simulink model "svm_test"  (Simulink 8.6)
settings: Solver=ode1  StartTime=0.0  StopTime=svm.tsim  FixedStep=uavsim.svm.tsample_model  RelTol=1e-3
values from neighbouring files (symbols this model uses):
  uavsim = loaded.uavsim    [svm_sandbox.m]
undefined symbols (not defined in the file or in its folder): svm
libraries: dspsrcs4 x2, aerolibtransform2 x2, aerolibanimutils x1, svm_lib x1, uavsimBlockset_UAV3DInterface x1
settings Model: Creator=j.bolting  LastModifiedBy=j.bolting
settings SolverCC: AutoInsertRateTranBlk=on
settings DataIOCC: SaveFormat=Dataset  SignalLoggingSaveFormat=Dataset
settings OptimizationCC: ExpressionDepthLimit=128
settings DebuggingCC: UnderspecifiedInitializationDetection=Simplified  MergeDetectMultiDrivingBlocksExec=error  SolverPrmCheckMsg=none  FcnCallInpInsideContextMsg=EnableAllAsError  StateNameClashWarn=none
settings HardwareCC: ProdBitPerPointer=64  ProdLargestAtomicFloat=Float  ProdIntDivRoundTo=Zero  ProdEndianess=LittleEndian  ProdWordSize=64  ProdHWDeviceType=Intel->x86-64 (Windows64)
settings GRTTargetCC: GeneratePreprocessorConditionals=Use local settings  CombineOutputUpdateFcns=on  GRTInterface=off
settings ConfigComp: CovModelRefEnable=off

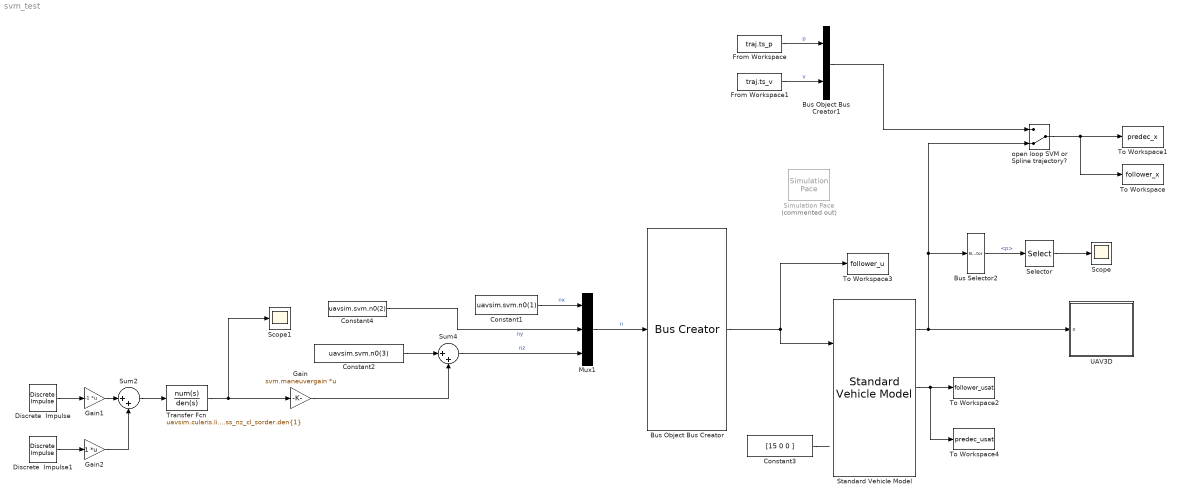
== system svm_test ==
  Bus Selector2 : BusSelector  OutputSignals=p
  Bus Object Bus Creator : BusCreator  Inputs=1  OutDataTypeStr=Bus: svm_bus_u  mask(BUS OBJECT Bus Creator){busType=Bus: svm_bus_u}
      mask prompts: busType "Bus Type"
      mask help:
      | Provides users the cabability to painlessly, instantly customize bus creators of output data type 'Bus:' by selecting the bus object type from a drop down menu dynamically populated by bus objects in the workspace.
      |
      | After pressing the "Apply Selection" button signal lines into the creator are populated and named with the elements in the chosen bus saving the user from having to recall and fill out signal line names.
      |
      | NOTE that when copying a Bus Object Bus Creator from your locked Library the link to the Library is automatically broken. This saves the user from having to Unlock Links To Library (From the Library menu.), Disable Link and finally Break Link (Both from the Model menu.) for every placed instance of the block.
      settings: AttributesFormatString=%<OutDataTypeStr>  CopyFcn=set_param(gcb, 'LinkStatus', 'none')
      mask TypeOptions busType: Bus: Acceleration | Bus: Aero | Bus: Airframe | Bus: Attitude | Bus: CMD | Bus: Environment | Bus: FlightGearData | Bus: Kinematics | Bus: Position | Bus: RotationalAcceleration | Bus: RotationalVelocity | Bus: Velocity | Bus: svm_bus_d_exo | Bus: svm_bus_u | Bus: svm_bus_x | Bus: svm_bus_xi
      mask Callback busType:
      | % Using variable names terminated with "_BOBC" to lessen the chances of
      | % collisions with existing workspace variables.
      | 
      | % Get the current block handle and mask handle.
      | handleCreator_BOBC = gcbh;
      | maskObj_BOBC       = Simulink.Mask.get(gcb);
      | 
      | % Get a list of variables in the workspace in order to search for the '1x1
      | % Bus' types.
      | wsVars_BOBC = whos;
      | 
      | % Reset the 'TypeOptions' bus list in case some '1x1 Bus' types have been
      | % deleted from or added to the workspace.
      | maskObj_BOBC.Parameters.TypeOptions = {'<empty>'};
      | 
      | % Reset the bus count.
      | busCount_BOBC = 0;
      | 
      | for index_BOBC = 1:length(wsVars_BOBC)
      | 
      |    % If the variable is a bus object...
      |    if strcmp(wsVars_BOBC(index_BOBC).class, 'Simulink.Bus')
      | 
      |       busCount_BOBC = busCount_BOBC + 1;
      | 
      |       % ... add it to the TypeOptions of the mask.
      |       maskObj_BOBC.Parameters.TypeOptions(busCount_BOBC) = ...
      |                                                            ...
      |                                  {['Bus: ', wsVars_BOBC(index_BOBC).name]};
      |    end
      | end
      | 
      | if busCount_BOBC == 0
      | 
      |    % If there are NO bus objects in the workspace then provide a warning
      |    % popup...
      |    warndlg('There are currently no bus objects in the workspace - you have no use for this block. Use a normal Bus Creator instead.')
      | 
      |    % ... and do nothing.
      | elseif ~strcmp(get_param(handleCreator_BOBC, 'OutDataTypeStr'), 'Inherit: auto')
      | 
      |    % If the currently selected bus data type ('OutDataTypeStr') is not
      |    % 'Inherit: auto' (i.e., if we are reopening the mask.) then get the
      |    % current 'OutDataTypeStr' and 'maskVal.' ('maskVal' is the selected
      |    % 'TypeOptions' list member.)
      |    outDatStr_BOBC = get_param(handleCreator_BOBC, 'OutDataTypeStr');
      |    maskVal_BOBC   = get_param(handleCreator_BOBC, 'MaskValues');
      | 
      |    if ~strcmp(outDatStr_BOBC, maskVal_BOBC{1})
      | 
      |       % Upon re-opening the mask if the default 'TypeOptions' list member
      |       % (The first one.) contained in 'maskVal' does not match the
      |       % currently selected bus data type ('OutDataTypeStr') then set the
      |       % 'TypeOptions' list member to the selected bus data type. (Cuts down
      |       % on confusion to have the displayed list member match the selected
      |       % bus data type rather than the first entry.)
      |       set_param(handleCreator_BOBC, 'MaskValues', {outDatStr_BOBC});
      |    end
      | end
      | 
      | % Clean up the workspace.
      | clear  handleCreator_BOBC  maskObj_BOBC     wsVars_BOBC ...
      |             busCount_BOBC    index_BOBC  outDatStr_BOBC ...
      |              maskVal_BOBC
      mask DialogControl applyMOCBSelection Prompt: Apply Selection
      mask DialogControl applyMOCBSelection Callback:
      | % Using variable names terminated with "_BOBC" to lessen the chances of
      | % collisions with existing workspace variables.
      | 
      | % Get the current block, current block handle and mask handle.
      | currentBlock_BOBC  = gcb;
      | handleCreator_BOBC = gcbh;
      | 
      | % Get the desired bus type...
      | desiredBusType_BOBC = get_param(handleCreator_BOBC, 'busType');
      | 
      | % ... and set the 'OutDataTypeStr' to it.
      | set_param(handleCreator_BOBC, 'OutDataTypeStr', desiredBusType_BOBC);
      | 
      | %% First delete any existing lines on the port.
      | % Get the line handles.
      | lh_BOBC = get_param(handleCreator_BOBC, 'LineHandles');
      | 
      | % If any lines exist (Non- -1 line handles.), delete them and start over.
      | if max(lh_BOBC.Inport > 0)
      | 
      |    for index_BOBC = 1:length(lh_BOBC.Inport)
      | 
      |       if lh_BOBC.Inport(index_BOBC) > 0
      | 
      |          delete_line(lh_BOBC.Inport(index_BOBC))
      |       end
      |    end
      | end
      | 
      | %% Then work on adding new lines.
      | 
      | % Get the block path for 'add_line' function.
      | blockPath_BOBC = get_param(handleCreator_BOBC, 'Parent');
      | 
      | % Get the newly selected bus type ('OutDataTypeStr')...
      | mocbBusType_BOBC = get_param(currentBlock_BOBC, 'OutDataTypeStr');
      | 
      | % ... and parse off "Bus: " so the string of the desired bus contained in
      | % 'OutDataTypeStr' matches the raw workspace bus names.
      | mocbBusType_BOBC = mocbBusType_BOBC(6:end);
      | 
      | % Then evaluate the string containing the workspace bus name which will
      | % load the desired bus parameters.
      | busParams_BOBC = eval(mocbBusType_BOBC);
      | 
      | % From the parameters grab the number of lines to add.
      | numLines_BOBC = length(busParams_BOBC.Elements);
      | 
      | % Set the number of inputs of the masked bus creator to the number of lines
      | % to add.
      | set_param(handleCreator_BOBC, 'Inputs', num2str(numLines_BOBC));
      | 
      | % Get (Inputs.) port handles so we can grab the positions of them.
      | ph_BOBC = get_param(handleCreator_BOBC, 'PortHandles');
      | 
      | for index_BOBC = 1:numLines_BOBC
      | 
      |    % Get the position of input port number 'index_BOBC'.
      |    portPos_BOBC = get_param(ph_BOBC.Inport(index_BOBC), 'Position');
      | 
      |    % Add a line from 50 pixels left of the port position to the port
      |    % position. (This must be done because it's the lines that get named,
      |    % not the port positions.)
      |    portLine_BOBC = add_line(blockPath_BOBC, [portPos_BOBC - [50 0]; portPos_BOBC]);
      | 
      |    % Rename the new line to the bus 'index_BOBC-st/nd/rd/th' element name.
      |    set_param(portLine_BOBC, 'Name', busParams_BOBC.Elements(index_BOBC).Name)
      | end
      | 
      | %% Cleanup the workspace.
      | clear    currentBlock_BOBC  handleCreator_BOBC      index_BOBC ...
      |        desiredBusType_BOBC             lh_BOBC  blockPath_BOBC ...
      |           mocbBusType_BOBC      busParams_BOBC   numLines_BOBC ...
      |                    ph_BOBC        portPos_BOBC   portLine_BOBC
  Bus Object Bus Creator1 : BusCreator  Inputs=2  OutDataTypeStr=Bus: svm_bus_x  mask(BUS OBJECT Bus Creator){busType=Bus: svm_bus_x}
      mask prompts: busType "Bus Type"
      mask help:
      | Provides users the cabability to painlessly, instantly customize bus creators of output data type 'Bus:' by selecting the bus object type from a drop down menu dynamically populated by bus objects in the workspace.
      |
      | After pressing the "Apply Selection" button signal lines into the creator are populated and named with the elements in the chosen bus saving the user from having to recall and fill out signal line names.
      |
      | NOTE that when copying a Bus Object Bus Creator from your locked Library the link to the Library is automatically broken. This saves the user from having to Unlock Links To Library (From the Library menu.), Disable Link and finally Break Link (Both from the Model menu.) for every placed instance of the block.
      settings: AttributesFormatString=%<OutDataTypeStr>  CopyFcn=set_param(gcb, 'LinkStatus', 'none')
      mask TypeOptions busType: Bus: Acceleration | Bus: Aero | Bus: Airframe | Bus: Attitude | Bus: CMD | Bus: Environment | Bus: FlightGearData | Bus: Kinematics | Bus: Position | Bus: RotationalAcceleration | Bus: RotationalVelocity | Bus: Velocity | Bus: svm_bus_d_exo | Bus: svm_bus_u | Bus: svm_bus_x | Bus: svm_bus_xi
      mask Callback busType:
      | % Using variable names terminated with "_BOBC" to lessen the chances of
      | % collisions with existing workspace variables.
      | 
      | % Get the current block handle and mask handle.
      | handleCreator_BOBC = gcbh;
      | maskObj_BOBC       = Simulink.Mask.get(gcb);
      | 
      | % Get a list of variables in the workspace in order to search for the '1x1
      | % Bus' types.
      | wsVars_BOBC = whos;
      | 
      | % Reset the 'TypeOptions' bus list in case some '1x1 Bus' types have been
      | % deleted from or added to the workspace.
      | maskObj_BOBC.Parameters.TypeOptions = {'<empty>'};
      | 
      | % Reset the bus count.
      | busCount_BOBC = 0;
      | 
      | for index_BOBC = 1:length(wsVars_BOBC)
      | 
      |    % If the variable is a bus object...
      |    if strcmp(wsVars_BOBC(index_BOBC).class, 'Simulink.Bus')
      | 
      |       busCount_BOBC = busCount_BOBC + 1;
      | 
      |       % ... add it to the TypeOptions of the mask.
      |       maskObj_BOBC.Parameters.TypeOptions(busCount_BOBC) = ...
      |                                                            ...
      |                                  {['Bus: ', wsVars_BOBC(index_BOBC).name]};
      |    end
      | end
      | 
      | if busCount_BOBC == 0
      | 
      |    % If there are NO bus objects in the workspace then provide a warning
      |    % popup...
      |    warndlg('There are currently no bus objects in the workspace - you have no use for this block. Use a normal Bus Creator instead.')
      | 
      |    % ... and do nothing.
      | elseif ~strcmp(get_param(handleCreator_BOBC, 'OutDataTypeStr'), 'Inherit: auto')
      | 
      |    % If the currently selected bus data type ('OutDataTypeStr') is not
      |    % 'Inherit: auto' (i.e., if we are reopening the mask.) then get the
      |    % current 'OutDataTypeStr' and 'maskVal.' ('maskVal' is the selected
      |    % 'TypeOptions' list member.)
      |    outDatStr_BOBC = get_param(handleCreator_BOBC, 'OutDataTypeStr');
      |    maskVal_BOBC   = get_param(handleCreator_BOBC, 'MaskValues');
      | 
      |    if ~strcmp(outDatStr_BOBC, maskVal_BOBC{1})
      | 
      |       % Upon re-opening the mask if the default 'TypeOptions' list member
      |       % (The first one.) contained in 'maskVal' does not match the
      |       % currently selected bus data type ('OutDataTypeStr') then set the
      |       % 'TypeOptions' list member to the selected bus data type. (Cuts down
      |       % on confusion to have the displayed list member match the selected
      |       % bus data type rather than the first entry.)
      |       set_param(handleCreator_BOBC, 'MaskValues', {outDatStr_BOBC});
      |    end
      | end
      | 
      | % Clean up the workspace.
      | clear  handleCreator_BOBC  maskObj_BOBC     wsVars_BOBC ...
      |             busCount_BOBC    index_BOBC  outDatStr_BOBC ...
      |              maskVal_BOBC
      mask DialogControl applyMOCBSelection Prompt: Apply Selection
      mask DialogControl applyMOCBSelection Callback:
      | % Using variable names terminated with "_BOBC" to lessen the chances of
      | % collisions with existing workspace variables.
      | 
      | % Get the current block, current block handle and mask handle.
      | currentBlock_BOBC  = gcb;
      | handleCreator_BOBC = gcbh;
      | 
      | % Get the desired bus type...
      | desiredBusType_BOBC = get_param(handleCreator_BOBC, 'busType');
      | 
      | % ... and set the 'OutDataTypeStr' to it.
      | set_param(handleCreator_BOBC, 'OutDataTypeStr', desiredBusType_BOBC);
      | 
      | %% First delete any existing lines on the port.
      | % Get the line handles.
      | lh_BOBC = get_param(handleCreator_BOBC, 'LineHandles');
      | 
      | % If any lines exist (Non- -1 line handles.), delete them and start over.
      | if max(lh_BOBC.Inport > 0)
      | 
      |    for index_BOBC = 1:length(lh_BOBC.Inport)
      | 
      |       if lh_BOBC.Inport(index_BOBC) > 0
      | 
      |          delete_line(lh_BOBC.Inport(index_BOBC))
      |       end
      |    end
      | end
      | 
      | %% Then work on adding new lines.
      | 
      | % Get the block path for 'add_line' function.
      | blockPath_BOBC = get_param(handleCreator_BOBC, 'Parent');
      | 
      | % Get the newly selected bus type ('OutDataTypeStr')...
      | mocbBusType_BOBC = get_param(currentBlock_BOBC, 'OutDataTypeStr');
      | 
      | % ... and parse off "Bus: " so the string of the desired bus contained in
      | % 'OutDataTypeStr' matches the raw workspace bus names.
      | mocbBusType_BOBC = mocbBusType_BOBC(6:end);
      | 
      | % Then evaluate the string containing the workspace bus name which will
      | % load the desired bus parameters.
      | busParams_BOBC = eval(mocbBusType_BOBC);
      | 
      | % From the parameters grab the number of lines to add.
      | numLines_BOBC = length(busParams_BOBC.Elements);
      | 
      | % Set the number of inputs of the masked bus creator to the number of lines
      | % to add.
      | set_param(handleCreator_BOBC, 'Inputs', num2str(numLines_BOBC));
      | 
      | % Get (Inputs.) port handles so we can grab the positions of them.
      | ph_BOBC = get_param(handleCreator_BOBC, 'PortHandles');
      | 
      | for index_BOBC = 1:numLines_BOBC
      | 
      |    % Get the position of input port number 'index_BOBC'.
      |    portPos_BOBC = get_param(ph_BOBC.Inport(index_BOBC), 'Position');
      | 
      |    % Add a line from 50 pixels left of the port position to the port
      |    % position. (This must be done because it's the lines that get named,
      |    % not the port positions.)
      |    portLine_BOBC = add_line(blockPath_BOBC, [portPos_BOBC - [50 0]; portPos_BOBC]);
      | 
      |    % Rename the new line to the bus 'index_BOBC-st/nd/rd/th' element name.
      |    set_param(portLine_BOBC, 'Name', busParams_BOBC.Elements(index_BOBC).Name)
      | end
      | 
      | %% Cleanup the workspace.
      | clear    currentBlock_BOBC  handleCreator_BOBC      index_BOBC ...
      |        desiredBusType_BOBC             lh_BOBC  blockPath_BOBC ...
      |           mocbBusType_BOBC      busParams_BOBC   numLines_BOBC ...
      |                    ph_BOBC        portPos_BOBC   portLine_BOBC
  Constant1 : Constant  Value=uavsim.svm.n0(1)
  Constant2 : Constant  Value=uavsim.svm.n0(3)
  Constant3 : Constant  Value=[15 0 0 ]
  Constant4 : Constant  Value=uavsim.svm.n0(2)
  Discrete  Impulse : dspsrcs4/Discrete  Impulse  Delay=10  SampleTime=1  FrameSample=1  OutputFrames=off  dataType=double  isSigned=on  wordLen=16  udDataType=sfix(16)  fracBitsMode=Best precision  numFracBits=15  OutDataTypeStr=double  LastOutDataTypeStr=double
  Discrete  Impulse1 : dspsrcs4/Discrete  Impulse  Delay=11  SampleTime=1  FrameSample=1  OutputFrames=off  dataType=double  isSigned=on  wordLen=16  udDataType=sfix(16)  fracBitsMode=Best precision  numFracBits=15  OutDataTypeStr=double  LastOutDataTypeStr=double
  From Workspace : FromWorkspace  VariableName=traj.ts_p  SampleTime=0
  From Workspace1 : FromWorkspace  VariableName=traj.ts_v  SampleTime=0
  Gain : Gain  Gain=svm.maneuvergain  Multiplication=Matrix(K*u)
  Gain1 : Gain  Gain=-1  Multiplication=Matrix(K*u)
  Gain2 : Gain  Multiplication=Matrix(K*u)
  Mux1 : Mux  Inputs=3
  Scope : Scope
  Scope1 : Scope
  Selector : Selector  InputPortWidth=3  IndexOptions=Index vector (dialog)  Indices=3  OutputSizes=1
  Simulation Pace : aerolibanimutils/Simulation Pace  Commented=on  SimulationPace=1  SleepMode=MATLAB Thread  OutputPaceError=on  SampleTime=1/25
      settings: AttributesFormatString=%<SimulationPace> sec/sec
  Standard Vehicle Model : svm_lib/Standard Vehicle Model  mask_p0_NED=[0 0 -50]  mask_v0_NED=svm.v0
  Sum2 : Sum  Inputs=|++
  Sum4 : Sum  Inputs=|++
  To Workspace : ToWorkspace  VariableName=follower_x  SaveFormat=Timeseries  SampleTime=-1
  To Workspace1 : ToWorkspace  VariableName=predec_x  SaveFormat=Timeseries  SampleTime=-1
  To Workspace2 : ToWorkspace  VariableName=follower_usat  SaveFormat=Timeseries  SampleTime=-1
  To Workspace3 : ToWorkspace  VariableName=follower_u  SaveFormat=Timeseries  SampleTime=-1
  To Workspace4 : ToWorkspace  VariableName=predec_usat  SaveFormat=Timeseries  SampleTime=-1
  Transfer Fcn : TransferFcn  Numerator=uavsim.cularis.linearModels.eulers.ss_nz_cl_sorder.num{1}  Denominator=uavsim.cularis.linearModels.eulers.ss_nz_cl_sorder.den{1}
  UAV3D : Subsystem
  open loop SVM or Spline trajectory? : ManualSwitch  CurrentSetting=0
  wires:
  Standard Vehicle Model/1 -> UAV3D/1(x), open loop SVM or Spline trajectory?/2, Bus Selector2/1
  Bus Object Bus Creator/1 -> To Workspace3/1, Standard Vehicle Model/1
  Gain/1 -> Sum4/2
  Constant2/1 -> Sum4/1
  Constant3/1 -> ?
  Bus Selector2/1 -> Selector/1  "<p>"
  Selector/1 -> Scope/1
  Sum4/1 -> Mux1/3  "nz"
  Constant1/1 -> Mux1/1  "nx"
  Constant4/1 -> Mux1/2  "ny"
  Sum2/1 -> Transfer Fcn/1
  Transfer Fcn/1 -> Gain/1, Scope1/1
  Standard Vehicle Model/2 -> To Workspace4/1, To Workspace2/1
  Discrete  Impulse/1 -> Gain1/1
  Discrete  Impulse1/1 -> Gain2/1
  Gain1/1 -> Sum2/1
  Gain2/1 -> Sum2/2
  From Workspace/1 -> Bus Object Bus Creator1/1  "p"
  From Workspace1/1 -> Bus Object Bus Creator1/2  "v"
  Bus Object Bus Creator1/1 -> open loop SVM or Spline trajectory?/1
  open loop SVM or Spline trajectory?/1 -> To Workspace/1, To Workspace1/1
  Mux1/1 -> Bus Object Bus Creator/1  "n"

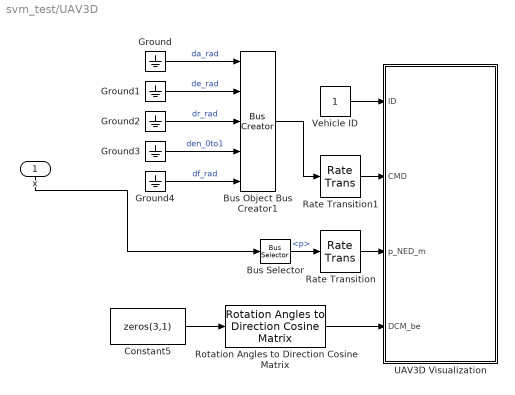
== system svm_test/UAV3D ==
  x : Inport
  Bus Selector : BusSelector  OutputSignals=p
  Bus Object Bus Creator1 : BusCreator  Inputs=5  OutDataTypeStr=Bus: CMD  mask(BUS OBJECT Bus Creator){busType=Bus: CMD}
      mask prompts: busType "Bus Type"
      mask help:
      | Provides users the cabability to painlessly, instantly customize bus creators of output data type 'Bus:' by selecting the bus object type from a drop down menu dynamically populated by bus objects in the workspace.
      |
      | After pressing the "Apply Selection" button signal lines into the creator are populated and named with the elements in the chosen bus saving the user from having to recall and fill out signal line names.
      |
      | NOTE that when copying a Bus Object Bus Creator from your locked Library the link to the Library is automatically broken. This saves the user from having to Unlock Links To Library (From the Library menu.), Disable Link and finally Break Link (Both from the Model menu.) for every placed instance of the block.
      settings: AttributesFormatString=%<OutDataTypeStr>  CopyFcn=set_param(gcb, 'LinkStatus', 'none')
      mask TypeOptions busType: Bus: Acceleration | Bus: Aero | Bus: Airframe | Bus: Attitude | Bus: CMD | Bus: Environment | Bus: FlightGearData | Bus: Kinematics | Bus: Position | Bus: RotationalAcceleration | Bus: RotationalVelocity | Bus: Velocity | Bus: svm_bus_d_exo | Bus: svm_bus_u | Bus: svm_bus_x | Bus: svm_bus_xi
      mask Callback busType:
      | % Using variable names terminated with "_BOBC" to lessen the chances of
      | % collisions with existing workspace variables.
      | 
      | % Get the current block handle and mask handle.
      | handleCreator_BOBC = gcbh;
      | maskObj_BOBC       = Simulink.Mask.get(gcb);
      | 
      | % Get a list of variables in the workspace in order to search for the '1x1
      | % Bus' types.
      | wsVars_BOBC = whos;
      | 
      | % Reset the 'TypeOptions' bus list in case some '1x1 Bus' types have been
      | % deleted from or added to the workspace.
      | maskObj_BOBC.Parameters.TypeOptions = {'<empty>'};
      | 
      | % Reset the bus count.
      | busCount_BOBC = 0;
      | 
      | for index_BOBC = 1:length(wsVars_BOBC)
      | 
      |    % If the variable is a bus object...
      |    if strcmp(wsVars_BOBC(index_BOBC).class, 'Simulink.Bus')
      | 
      |       busCount_BOBC = busCount_BOBC + 1;
      | 
      |       % ... add it to the TypeOptions of the mask.
      |       maskObj_BOBC.Parameters.TypeOptions(busCount_BOBC) = ...
      |                                                            ...
      |                                  {['Bus: ', wsVars_BOBC(index_BOBC).name]};
      |    end
      | end
      | 
      | if busCount_BOBC == 0
      | 
      |    % If there are NO bus objects in the workspace then provide a warning
      |    % popup...
      |    warndlg('There are currently no bus objects in the workspace - you have no use for this block. Use a normal Bus Creator instead.')
      | 
      |    % ... and do nothing.
      | elseif ~strcmp(get_param(handleCreator_BOBC, 'OutDataTypeStr'), 'Inherit: auto')
      | 
      |    % If the currently selected bus data type ('OutDataTypeStr') is not
      |    % 'Inherit: auto' (i.e., if we are reopening the mask.) then get the
      |    % current 'OutDataTypeStr' and 'maskVal.' ('maskVal' is the selected
      |    % 'TypeOptions' list member.)
      |    outDatStr_BOBC = get_param(handleCreator_BOBC, 'OutDataTypeStr');
      |    maskVal_BOBC   = get_param(handleCreator_BOBC, 'MaskValues');
      | 
      |    if ~strcmp(outDatStr_BOBC, maskVal_BOBC{1})
      | 
      |       % Upon re-opening the mask if the default 'TypeOptions' list member
      |       % (The first one.) contained in 'maskVal' does not match the
      |       % currently selected bus data type ('OutDataTypeStr') then set the
      |       % 'TypeOptions' list member to the selected bus data type. (Cuts down
      |       % on confusion to have the displayed list member match the selected
      |       % bus data type rather than the first entry.)
      |       set_param(handleCreator_BOBC, 'MaskValues', {outDatStr_BOBC});
      |    end
      | end
      | 
      | % Clean up the workspace.
      | clear  handleCreator_BOBC  maskObj_BOBC     wsVars_BOBC ...
      |             busCount_BOBC    index_BOBC  outDatStr_BOBC ...
      |              maskVal_BOBC
      mask DialogControl applyMOCBSelection Prompt: Apply Selection
      mask DialogControl applyMOCBSelection Callback:
      | % Using variable names terminated with "_BOBC" to lessen the chances of
      | % collisions with existing workspace variables.
      | 
      | % Get the current block, current block handle and mask handle.
      | currentBlock_BOBC  = gcb;
      | handleCreator_BOBC = gcbh;
      | 
      | % Get the desired bus type...
      | desiredBusType_BOBC = get_param(handleCreator_BOBC, 'busType');
      | 
      | % ... and set the 'OutDataTypeStr' to it.
      | set_param(handleCreator_BOBC, 'OutDataTypeStr', desiredBusType_BOBC);
      | 
      | %% First delete any existing lines on the port.
      | % Get the line handles.
      | lh_BOBC = get_param(handleCreator_BOBC, 'LineHandles');
      | 
      | % If any lines exist (Non- -1 line handles.), delete them and start over.
      | if max(lh_BOBC.Inport > 0)
      | 
      |    for index_BOBC = 1:length(lh_BOBC.Inport)
      | 
      |       if lh_BOBC.Inport(index_BOBC) > 0
      | 
      |          delete_line(lh_BOBC.Inport(index_BOBC))
      |       end
      |    end
      | end
      | 
      | %% Then work on adding new lines.
      | 
      | % Get the block path for 'add_line' function.
      | blockPath_BOBC = get_param(handleCreator_BOBC, 'Parent');
      | 
      | % Get the newly selected bus type ('OutDataTypeStr')...
      | mocbBusType_BOBC = get_param(currentBlock_BOBC, 'OutDataTypeStr');
      | 
      | % ... and parse off "Bus: " so the string of the desired bus contained in
      | % 'OutDataTypeStr' matches the raw workspace bus names.
      | mocbBusType_BOBC = mocbBusType_BOBC(6:end);
      | 
      | % Then evaluate the string containing the workspace bus name which will
      | % load the desired bus parameters.
      | busParams_BOBC = eval(mocbBusType_BOBC);
      | 
      | % From the parameters grab the number of lines to add.
      | numLines_BOBC = length(busParams_BOBC.Elements);
      | 
      | % Set the number of inputs of the masked bus creator to the number of lines
      | % to add.
      | set_param(handleCreator_BOBC, 'Inputs', num2str(numLines_BOBC));
      | 
      | % Get (Inputs.) port handles so we can grab the positions of them.
      | ph_BOBC = get_param(handleCreator_BOBC, 'PortHandles');
      | 
      | for index_BOBC = 1:numLines_BOBC
      | 
      |    % Get the position of input port number 'index_BOBC'.
      |    portPos_BOBC = get_param(ph_BOBC.Inport(index_BOBC), 'Position');
      | 
      |    % Add a line from 50 pixels left of the port position to the port
      |    % position. (This must be done because it's the lines that get named,
      |    % not the port positions.)
      |    portLine_BOBC = add_line(blockPath_BOBC, [portPos_BOBC - [50 0]; portPos_BOBC]);
      | 
      |    % Rename the new line to the bus 'index_BOBC-st/nd/rd/th' element name.
      |    set_param(portLine_BOBC, 'Name', busParams_BOBC.Elements(index_BOBC).Name)
      | end
      | 
      | %% Cleanup the workspace.
      | clear    currentBlock_BOBC  handleCreator_BOBC      index_BOBC ...
      |        desiredBusType_BOBC             lh_BOBC  blockPath_BOBC ...
      |           mocbBusType_BOBC      busParams_BOBC   numLines_BOBC ...
      |                    ph_BOBC        portPos_BOBC   portLine_BOBC
  Constant5 : Constant  Value=zeros(3,1)
  Ground{,1..4} (5 alike) : Ground
  Rate Transition : RateTransition  OutPortSampleTime=1/25
  Rate Transition1 : RateTransition  OutPortSampleTime=1/25
  Rotation Angles to Direction Cosine Matrix : aerolibtransform2/Rotation Angles to Direction Cosine Matrix  rotationOrder=ZYX
  UAV3D Visualization : Subsystem  AncestorBlock=formationFlyingBlockset/UAV3D Visualization  TreatAsAtomicUnit=on  SystemSampleTime=1/25  mask{mask_visual=2}
      mask prompts: mask_visual "3D model"
      mask TypeOptions mask_visual: 0 | 1 | 2 | 3
  Vehicle ID : Constant
  wires:
  Ground1/1 -> Bus Object Bus Creator1/2  "de_rad"
  Ground4/1 -> Bus Object Bus Creator1/5  "df_rad"
  Rate Transition1/1 -> UAV3D Visualization/2(CMD)
  Ground3/1 -> Bus Object Bus Creator1/4  "den_0to1"
  Ground2/1 -> Bus Object Bus Creator1/3  "dr_rad"
  Ground/1 -> Bus Object Bus Creator1/1  "da_rad"
  Rotation Angles to Direction Cosine Matrix/1 -> UAV3D Visualization/4(DCM_be)
  Bus Object Bus Creator1/1 -> Rate Transition1/1
  Vehicle ID/1 -> UAV3D Visualization/1(ID)
  Bus Selector/1 -> Rate Transition/1  "<p>"
  Constant5/1 -> Rotation Angles to Direction Cosine Matrix/1
  Rate Transition/1 -> UAV3D Visualization/3(p_NED_m)
  x/1 -> Bus Selector/1

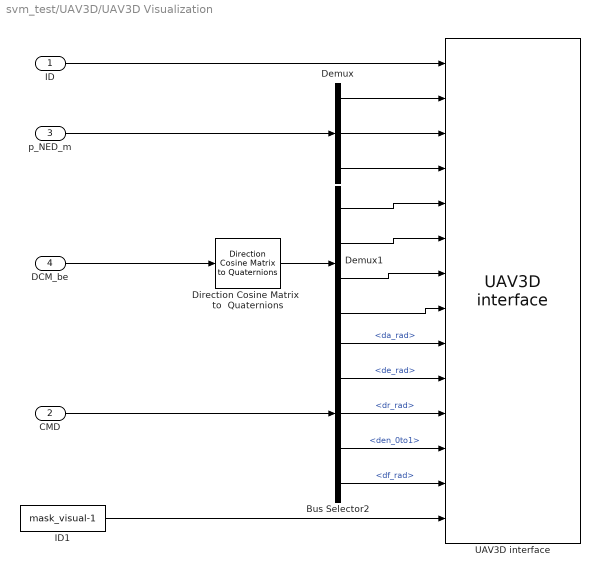
== system svm_test/UAV3D/UAV3D Visualization ==
  ID : Inport
  CMD : Inport  Port=2  OutDataTypeStr=Bus: CMD
  p_NED_m : Inport  Port=3
  DCM_be : Inport  Port=4
  Bus Selector2 : BusSelector  OutputSignals=da_rad,de_rad,dr_rad,den_0to1,df_rad
  Demux : Demux  Outputs=3
  Demux1 : Demux
  Direction Cosine Matrix   to  Quaternions : aerolibtransform2/Direction Cosine Matrix  to Quaternions
  ID1 : Constant  Value=mask_visual-1
  UAV3D interface : uavsimBlockset_UAV3DInterface/UAV3D interface  ip='localhost'  udpport=4445
  wires:
  Bus Selector2/5 -> UAV3D interface/13  "<df_rad>"
  Bus Selector2/4 -> UAV3D interface/12  "<den_0to1>"
  Bus Selector2/3 -> UAV3D interface/11  "<dr_rad>"
  Bus Selector2/2 -> UAV3D interface/10  "<de_rad>"
  Bus Selector2/1 -> UAV3D interface/9  "<da_rad>"
  CMD/1 -> Bus Selector2/1
  p_NED_m/1 -> Demux/1
  Demux/3 -> UAV3D interface/4
  Demux/2 -> UAV3D interface/3
  Demux/1 -> UAV3D interface/2
  DCM_be/1 -> Direction Cosine Matrix   to  Quaternions/1
  Demux1/1 -> UAV3D interface/5
  Demux1/2 -> UAV3D interface/6
  Demux1/3 -> UAV3D interface/7
  Demux1/4 -> UAV3D interface/8
  Direction Cosine Matrix   to  Quaternions/1 -> Demux1/1
  ID/1 -> UAV3D interface/1
  ID1/1 -> UAV3D interface/14
